simulink model "Ejercicio_1"  (R2021b)
settings: Solver=VariableStepAuto  StartTime=0.0  StopTime=inf  RelTol=1e-3
libraries: dspsrcs4 x4, simulink_extras x3, dsparch4 x2, commrandsrc3 x1
settings Model: Creator=Hagui  LastModifiedBy=Hagui

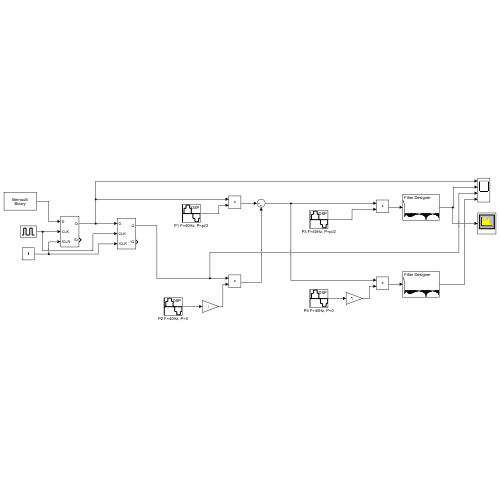
[thumbnail: Simulink's stored preview of the top-level diagram]
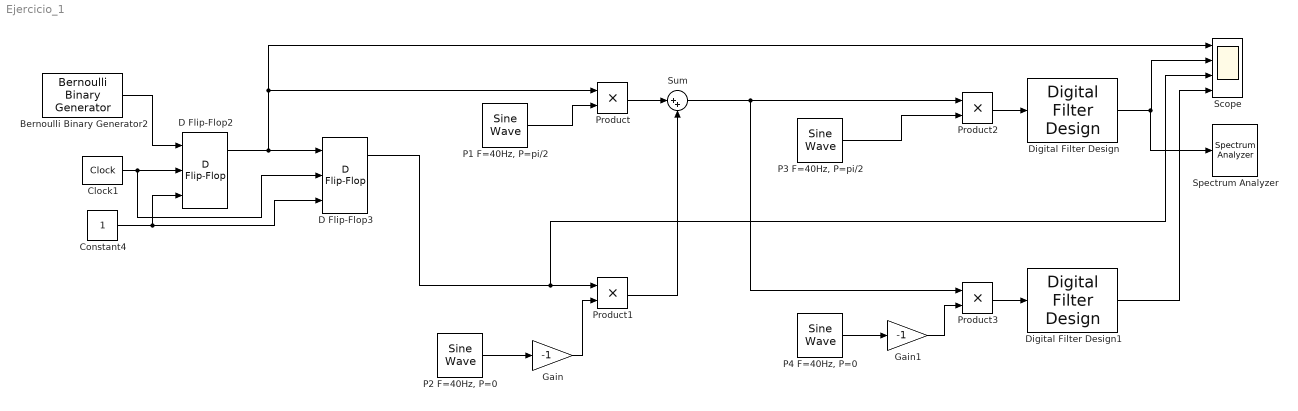
== system Ejercicio_1 ==
  Bernoulli Binary Generator2 : commrandsrc3/Bernoulli Binary Generator  ProbabilityOfZero=0.5  SeedSource=Auto  Seed=0  SampleTime=1  SamplesPerFrame=1  OutputDataType=boolean  SimulateUsing=Interpreted execution
  Clock1 : simulink_extras/Flip Flops/Clock  period=1
  Constant4 : Constant
  D Flip-Flop2 : simulink_extras/Flip Flops/D Flip-Flop
  D Flip-Flop3 : simulink_extras/Flip Flops/D Flip-Flop
  Digital Filter Design : dsparch4/Digital Filter Design  mwdsp_browser_bugfix_var=off
  Digital Filter Design1 : dsparch4/Digital Filter Design  mwdsp_browser_bugfix_var=off
  Gain : Gain  Gain=-1
  Gain1 : Gain  Gain=-1
  "P1 F=40Hz, P=pi/2" : dspsrcs4/Sine Wave  Amplitude=1  Frequency=40  Phase=pi/2  SampleMode=Discrete  OutComplex=Real  CompMethod=Trigonometric fcn  TableSize=Speed  SampleTime=1/1000  SamplesPerFrame=1  ResetState=Restart at time zero  OutputFrames=off  dataType=double  wordLen=16  udDataType=sfix(16)  fracBitsMode=Best precision  numFracBits=15  OutDataTypeStr=double  LastOutDataTypeStr=double
  "P2 F=40Hz, P=0" : dspsrcs4/Sine Wave  Amplitude=1  Frequency=40  Phase=0  SampleMode=Discrete  OutComplex=Real  CompMethod=Trigonometric fcn  TableSize=Speed  SampleTime=1/1000  SamplesPerFrame=1  ResetState=Restart at time zero  OutputFrames=off  dataType=double  wordLen=16  udDataType=sfix(16)  fracBitsMode=Best precision  numFracBits=15  OutDataTypeStr=double  LastOutDataTypeStr=double
  "P3 F=40Hz, P=pi/2" : dspsrcs4/Sine Wave  Amplitude=1  Frequency=40  Phase=pi/2  SampleMode=Discrete  OutComplex=Real  CompMethod=Trigonometric fcn  TableSize=Speed  SampleTime=1/1000  SamplesPerFrame=1  ResetState=Restart at time zero  OutputFrames=off  dataType=double  wordLen=16  udDataType=sfix(16)  fracBitsMode=Best precision  numFracBits=15  OutDataTypeStr=double  LastOutDataTypeStr=double
  "P4 F=40Hz, P=0" : dspsrcs4/Sine Wave  Amplitude=1  Frequency=40  Phase=0  SampleMode=Discrete  OutComplex=Real  CompMethod=Trigonometric fcn  TableSize=Speed  SampleTime=1/1000  SamplesPerFrame=1  ResetState=Restart at time zero  OutputFrames=off  dataType=double  wordLen=16  udDataType=sfix(16)  fracBitsMode=Best precision  numFracBits=15  OutDataTypeStr=double  LastOutDataTypeStr=double
  Product{,1..3} (4 alike) : Product
  Scope : Scope  NumInputPorts=4
  Spectrum Analyzer : SpectrumAnalyzer
  Sum : Sum  Inputs=|++
  wires:
  "P1 F=40Hz, P=pi/2"/1 -> Product/2
  "P2 F=40Hz, P=0"/1 -> Gain/1
  Gain/1 -> Product1/2
  Constant4/1 -> D Flip-Flop3/3, D Flip-Flop2/3
  Clock1/1 -> D Flip-Flop3/2, D Flip-Flop2/2
  D Flip-Flop2/1 -> Scope/1, Product/1, D Flip-Flop3/1
  Bernoulli Binary Generator2/1 -> D Flip-Flop2/1
  D Flip-Flop3/1 -> Scope/3, Product1/1
  Product/1 -> Sum/1
  Product1/1 -> Sum/2
  Product3/1 -> Digital Filter Design1/1
  Gain1/1 -> Product3/2
  "P4 F=40Hz, P=0"/1 -> Gain1/1
  "P3 F=40Hz, P=pi/2"/1 -> Product2/2
  Product2/1 -> Digital Filter Design/1
  Sum/1 -> Product3/1, Product2/1
  Digital Filter Design/1 -> Spectrum Analyzer/1, Scope/2
  Digital Filter Design1/1 -> Scope/4
